simulink model "RcsAnalysis"  (R2023b)
settings: Solver=VariableStepAuto  StartTime=0.0  StopTime=30  RelTol=1e-3
model workspace (MAT data in the model file):
  thrust = 2
libraries: simulink_extras x3
settings Model: Creator=Hoboness  LastModifiedBy=Hoboness

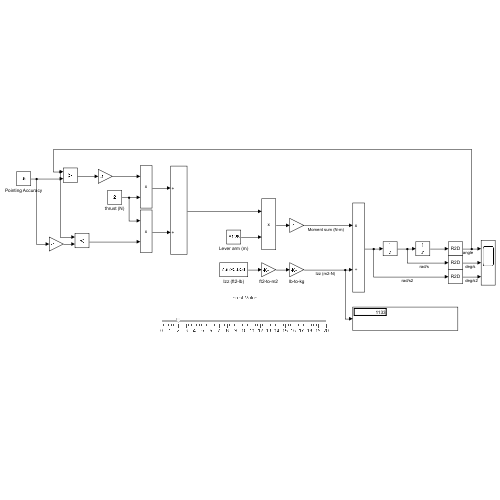
[thumbnail: Simulink's stored preview of the top-level diagram]
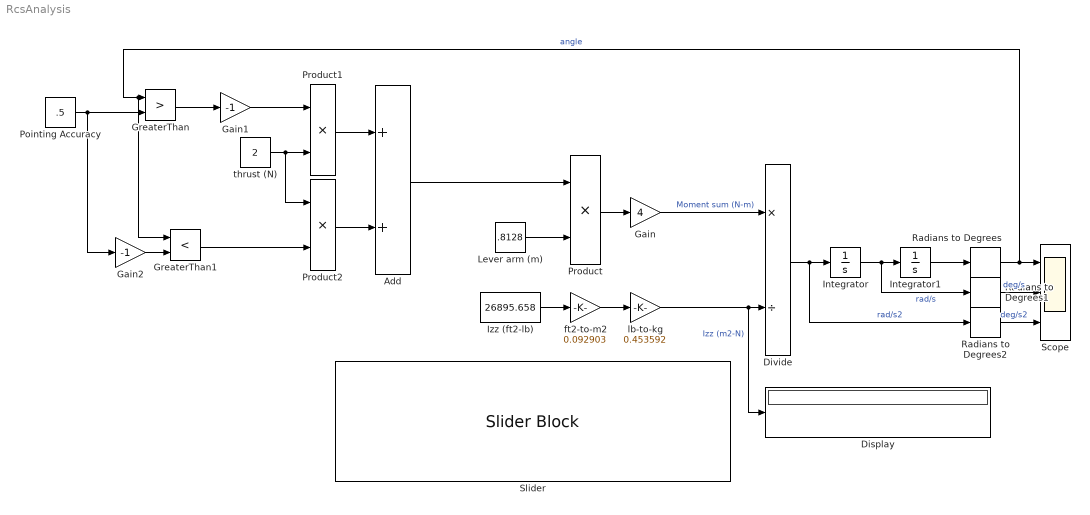
== system RcsAnalysis ==
  Add : Sum
  Display : Display
  Divide : Product  Inputs=*/
  Gain : Gain  Gain=4
  Gain1 : Gain  Gain=-1
  Gain2 : Gain  Gain=-1
  GreaterThan : RelationalOperator  Operator=>  OutDataTypeStr=boolean  RndMeth=Simplest  InputSameDT=off
  GreaterThan1 : RelationalOperator  Operator=<  OutDataTypeStr=boolean  RndMeth=Simplest  InputSameDT=off
  Integrator : Integrator
  Integrator1 : Integrator  InitialCondition=deg2rad(.51)
  Izz (ft2-lb) : Constant  Value=26895.658
  Lever arm (m) : Constant  Value=.8128
  Pointing Accuracy : Constant  Value=.5
  Product : Product
  Product1 : Product
  Product2 : Product
  Radians to Degrees : simulink_extras/Transformations/Radians to Degrees
  Radians to Degrees1 : simulink_extras/Transformations/Radians to Degrees
  Radians to Degrees2 : simulink_extras/Transformations/Radians to Degrees
  Scope : Scope  NumInputPorts=3
  Slider : SliderBlock  ScaleMax=20
  ft2-to-m2 : Gain  Gain=0.092903
  lb-to-kg : Gain  Gain=0.453592
  thrust (N) : Constant  Value=2
  wires:
  Izz (ft2-lb)/1 -> ft2-to-m2/1
  ft2-to-m2/1 -> lb-to-kg/1
  lb-to-kg/1 -> Display/1, Divide/2  "Izz (m2-N)"
  Lever arm (m)/1 -> Product/2
  thrust (N)/1 -> Product2/1, Product1/2
  Product/1 -> Gain/1
  Gain/1 -> Divide/1  "Moment sum (N-m)"
  Divide/1 -> Radians to Degrees2/1, Integrator/1  "rad/s2"
  Integrator/1 -> Radians to Degrees1/1, Integrator1/1  "rad/s"
  Integrator1/1 -> Radians to Degrees/1
  Radians to Degrees/1 -> GreaterThan1/1, GreaterThan/1, Scope/1  "angle"
  Pointing Accuracy/1 -> Gain2/1, GreaterThan/2
  GreaterThan/1 -> Gain1/1
  Gain1/1 -> Product1/1
  Gain2/1 -> GreaterThan1/2
  GreaterThan1/1 -> Product2/2
  Product1/1 -> Add/1
  Product2/1 -> Add/2
  Add/1 -> Product/1
  Radians to Degrees1/1 -> Scope/2  "deg/s"
  Radians to Degrees2/1 -> Scope/3  "deg/s2"
